simulink model "PID_accel_noise"  (R2021b)
settings: Solver=VariableStepAuto  StartTime=0.0  StopTime=2  RelTol=1e-3
undefined symbols (not defined in the file or in its folder): param
libraries: slpidlib x1, commchan3 x1
settings Model: Creator=Natalie  LastModifiedBy=Trevor

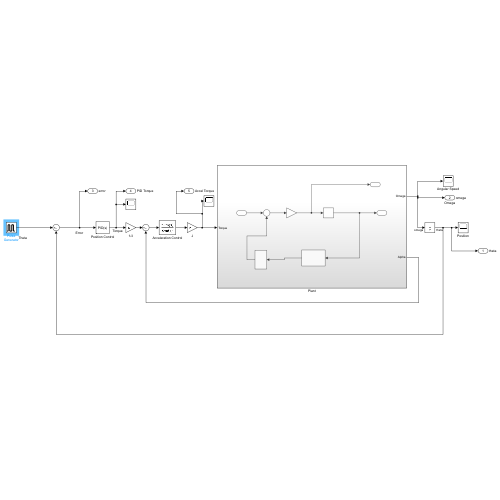
[thumbnail: Simulink's stored preview of the top-level diagram]
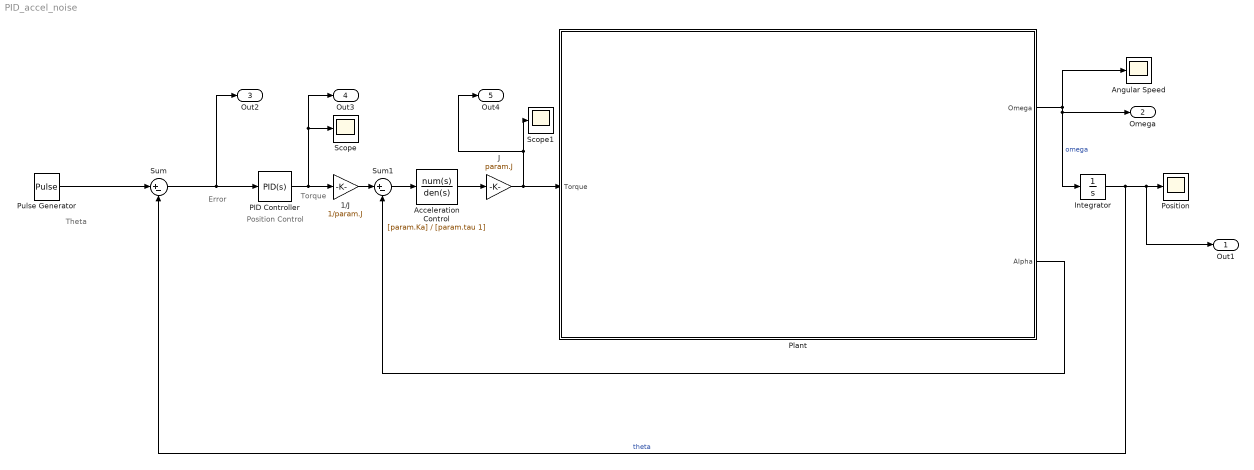
== system PID_accel_noise ==
  note: Position Control
  note: Torque
  note: Error
  note: Theta
  1/J : Gain  Gain=1/param.J
  Acceleration Control : TransferFcn  Numerator=[param.Ka]  Denominator=[param.tau 1]
  Angular Speed : Scope
  Integrator : Integrator
  J : Gain  Gain=param.J
  PID Controller : slpidlib/PID Controller  Controller=PID  Form=Parallel  TimeDomain=Continuous-time  UseExternalTs=off  SampleTime=-1  IntegratorMethod=Forward Euler  FilterMethod=Forward Euler  ControllerParametersSource=internal  P=param.Kp  I=param.Ki  D=param.Kd  UseFilter=on  N=param.N  TunerSelectOption=Transfer Function Based (PID Tuner App)  InitialConditionSource=internal  InitialConditionForIntegrator=0  InitialConditionForFilter=0  DifferentiatorICPrevScaledInput=0  ExternalReset=none  TrackingMode=off  Kt=1  LimitOutput=off  SatLimitsSource=internal  UpperSaturationLimit=inf  LowerSaturationLimit=-inf  LinearizeAsGain=on  AntiWindupMode=none  Kb=1  POutMin=[]  POutMax=[]  IOutMin=[]  IOutMax=[]  DOutMin=[]  DOutMax=[]  NOutMin=[]  NOutMax=[]  SumOutMin=[]  SumOutMax=[]  SaturationOutMin=[]  SaturationOutMax=[]  PParamMin=[]  PParamMax=[]  IParamMin=[]  IParamMax=[]  DParamMin=[]  DParamMax=[]  NParamMin=[]  NParamMax=[]  KbParamMin=[]  KbParamMax=[]  KtParamMin=[]  KtParamMax=[]  KbOutMin=[]  KbOutMax=[]  KtOutMin=[]  KtOutMax=[]  IntegratorOutMin=[]  IntegratorOutMax=[]  FilterOutMin=[]  FilterOutMax=[]  SumI1OutMin=[]  SumI1OutMax=[]  SumI2OutMin=[]  SumI2OutMax=[]  SumI3OutMin=[]  SumI3OutMax=[]  SumI4OutMin=[]  SumI4OutMax=[]  SumDOutMin=[]  SumDOutMax=[]  DifferentiatorOutMin=[]  DifferentiatorOutMax=[]  FilterDiffOutCoefMin=[]  FilterDiffOutCoefMax=[]  ReciprocalOutMin=[]  ReciprocalOutMax=[]  SumDenOutMin=[]  SumDenOutMax=[]  SumNumOutMin=[]  SumNumOutMax=[]  DivideOutMin=[]  DivideOutMax=[]  UdiffTsProdOutMin=[]  UdiffTsProdOutMax=[]  NTsProdOutMin=[]  NTsProdOutMax=[]  UintegralTsProdOutMin=[]  UintegralTsProdOutMax=[]  UngainTsProdOutMin=[]  UngainTsProdOutMax=[]  IntegratorContinuousStateAttributes=''  IntegratorStateMustResolveToSignalObject=off  IntegratorRTWStateStorageClass=Auto  FilterContinuousStateAttributes=''  FilterStateMustResolveToSignalObject=off  FilterRTWStateStorageClass=Auto  ParallelPVariant=InternalParameters  IdealPVariant=Disabled  IVariant=InternalParameters  DVariant=InternalParameters  IntegratorVariant=Continuous  SatVariant=Disabled  AWVariant=Passthrough  PCopyVariant=Disabled  TRVariant=Disabled  FdbkBlocksVariant=Forward  IdealPFdbkVariant=Disabled  SatFdbkVariant=Disabled  DerivativeFilterVariant=ContFilter  NVariant=InternalParameters  NCopyVariant=Disabled  FilterICVariant=InternalICsFilter  IntegratorICVariant=InternalICs  ExternalResetVariant=Disabled  TRSumVariant=Passthrough  SumFdbkVariant=Disabled  SumVariant=Sum_PID  TsampFilterVariant=InternalTs  TsampNgainVariant=Passthrough  TsampIntegralVariant=Passthrough  ExternalSaturationOutDataTypeStr=Inherit: Same as second input
  Plant : Subsystem
  Position : Scope
  Pulse Generator : DiscretePulseGenerator  PulseType=Time based  PulseWidth=50
  Scope : Scope
  Scope1 : Scope
  Sum : Sum  Inputs=|+-
  Sum1 : Sum  Inputs=|+-
  Out1 : Outport  SignalName=theta
  Omega : Outport  Port=2  SignalName=omega
  Out2 : Outport  Port=3  SignalName=error
  Out3 : Outport  Port=4  SignalName=PID Torque
  Out4 : Outport  Port=5  SignalName=Accel Torque
  wires:
  Plant/1(Omega) -> Integrator/1, Omega/1, Angular Speed/1  "omega"
  Integrator/1 -> Out1/1, Position/1, Sum/2  "theta"
  Pulse Generator/1 -> Sum/1
  Sum/1 -> Out2/1, PID Controller/1
  PID Controller/1 -> 1/J/1, Scope/1, Out3/1
  1/J/1 -> Sum1/1
  Plant/2(Alpha) -> Sum1/2
  J/1 -> Out4/1, Scope1/1, Plant/1(Torque)
  Sum1/1 -> Acceleration Control/1
  Acceleration Control/1 -> J/1

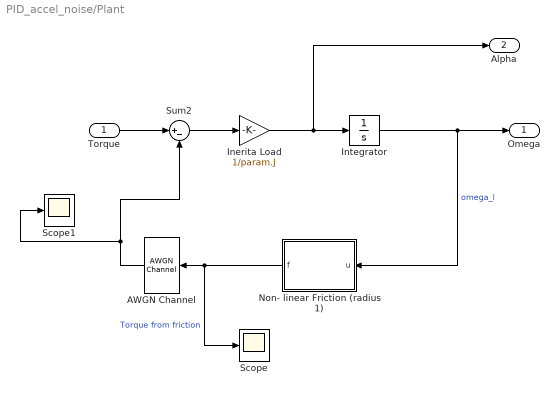
== system PID_accel_noise/Plant ==
  Torque : Inport
  AWGN Channel : commchan3/AWGN Channel  InputProcessing=Columns as channels (frame based)  seed=67  noiseMode=Variance from mask  EbNodB=10  EsNodB=10  SNRdB=10  bitsPerSym=1  Ps=1  Tsym=1  variance=0.001
  Inerita Load : Gain  Gain=1/param.J
  Integrator : Integrator
  Non- linear Friction (radius 1) : MATLAB Function  TreatAsAtomicUnit=on
  Scope : Scope
  Scope1 : Scope
  Sum2 : Sum  Inputs=|+-
  Omega : Outport
  Alpha : Outport  Port=2
  wires:
  Integrator/1 -> Omega/1, Non- linear Friction (radius 1)/1(u)  "omega_l"
  Torque/1 -> Sum2/1
  Sum2/1 -> Inerita Load/1
  Inerita Load/1 -> Alpha/1, Integrator/1
  Non- linear Friction (radius 1)/1(f) -> Scope/1, AWGN Channel/1  "Torque from friction"
  AWGN Channel/1 -> Scope1/1, Sum2/2

== matlab function PID_accel_noise/Plant/Non- linear Friction (radius 1) ==
  data: u input; f output; param parameter
function f = friction_m(u, param)

%FRICTION_M Nonlinear friction model with Stribeck, Coulomb and viscous

% dissipation effects.

% Output equation.

f = param.g1*(tanh(param.g2*u)-tanh(param.g3*u)) ... % Stribeck effect.
+ param.g4*tanh(param.g5*u) ... % Coulomb effect.
+ param.g6*u; % Viscous dissipation term.

end
